simulink model "myStateFlow"  (R2018b)
settings: Solver=FixedStepAuto  StartTime=0.0  StopTime=2555  FixedStep=Ts  RelTol=1e-3
undefined symbols (not defined in the file or in its folder): DiscIntNeverNeededParam, plannedpath, pos0, posf
libraries: simulink x3
(part 2 of 2)

== matlab function myStateFlow/Navigator/Switch Case Action Subsystem2/MATLAB Function2 ==
  data: data input; dataout output; sizedata input
function dataout = fcn(data,sizedata)
dataout = zeros(1,size(sizedata,1));
for i = 1:size(sizedata,1)
    dataout(1,i) = data;
end

== matlab function myStateFlow/Navigator/Switch Case Action Subsystem2/MATLAB Function3 ==
  data: data input; dataout output; sizedata input
function dataout = fcn(data,sizedata)
dataout = zeros(size(sizedata));
dataout(1,:) = data;
